simulink library "lib_electric_machine2"  (Simulink 10.1)
settings: Solver=VariableStepAuto  StartTime=0.0  StopTime=10.0  RelTol=1e-3
undefined symbols (not defined in the file or in its folder): amb_tmp, fd_ratio, gb_ratio, gc_inertia, gc_map_spd, gc_map_trq, gc_max_crrnt, gc_max_trq, gc_outpwr_map, gc_overtrq_factor, gc_spd_scale, gc_trq_scale, mc_cp, mc_inertia, mc_init_tmp, mc_inpwr_map, mc_map_spd, mc_map_trq, mc_mass, mc_max_crrnt, mc_max_gen_trq, mc_max_trq, mc_overtrq_factor, mc_sarea, mc_spd_scale, mc_th_calc, mc_trq_scale, mc_tstat, veh_mass, wh_radius
undefined symbols (not defined in the file): logFlag
libraries: lib_electric_machine x1
(part 1 of 3)
settings Model: Creator=sateeshk  LastModifiedBy=sateeshk
settings Model: ModifiedComment=|
  | mokeefe -- Thu Apr 18 08:27:13 2002 -- Version 1.18
  | saving the model:
  | o "without the model browser open"
  | o with only top-level screen visible
  | o with "fit to view" enabled
  | o with "status bar" off and "toolbar" off
  | o with "prompt to update model history with each save" on
settings Model: ModifiedHistory=|
  | mokeefe -- Thu Apr 18 08:27:13 2002 -- Version 1.18
  | saving the model:
  | o "without the model browser open"
  | o with only top-level screen visible
  | o with "fit to view" enabled
  | o with "status bar" off and "toolbar" off
  | o with "prompt to update model history with each save" on
  | 
  | mokeefe -- Thu Apr 18 08:27:13 2002 -- Version 1.18
  | saving the model:
  | o "without the model browser open"
  | o with only top-level screen visible
  | o with "fit to view" enabled
  | o with "status bar" off and "toolbar" off
  | o with "prompt to update model history with each save" on

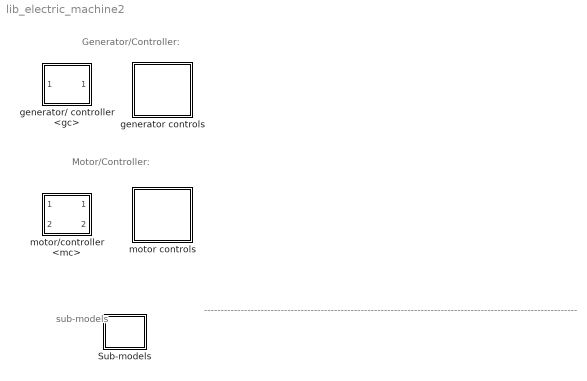
== system lib_electric_machine2 ==
  note: Generator/Controller:
  note: Motor/Controller:
  note: ----------------------------------------------------------------------------------------------------------------
  note: sub-models
  Sub-models : Subsystem
  generator controls : Subsystem
  generator/ controller <gc> : Subsystem  mask(Stand-Alone Generator/Controller Mask){generalName='gc', logPick=Log, initFileName={}, modCell={}, imgFileName='bdi_mc.jpg', DEBUG=OFF}
      mask prompts: generalName "General Name of this Component [char]"; logPick "Log Variables to Workspace?"; initFileName "Initialization File(s) [cell array of char]"; modCell "Modification Cell [2 column cell array of param and val]"; imgFileName "Icon image file name [char--evaluated]"
      mask init:
      | % initialization via m-file script
      | advSACompMaskInit;
      mask TypeOptions logPick: Don't Log | Log
      mask TypeOptions DEBUG: ON | OFF
      mask Display: image(imread(imgFileName))
  motor controls : Subsystem
  motor/controller <mc> : Subsystem  mask(Stand-Alone Motor/Controller Mask){generalName='mc', logPick=Log, initFileName={}, modCell={}, imgFileName='bdi_mc.jpg', DEBUG=OFF}
      mask prompts: generalName "General Name of this Component [char]"; logPick "Log Variables to Workspace?"; initFileName "Initialization File(s) [cell array of char]"; modCell "Modification Cell [2 column cell array of param and val]"; imgFileName "Icon image file name [char--evaluated]"
      mask init:
      | % initialization via m-file script
      | advSACompMaskInit;
      mask TypeOptions logPick: Don't Log | Log
      mask TypeOptions DEBUG: ON | OFF
      mask Display: image(imread(imgFileName))

== system lib_electric_machine2/Sub-models ==
  motor inertia as a function of total vehicle inertia (generous approximation) : Subsystem
  veh mass calc : Subsystem

== system lib_electric_machine2/generator controls ==

== system lib_electric_machine2/generator/ controller <gc> ==
  note: Generator/ CONTROLLER
      | Interface
  "torque and speed supplied to rotor (Nm), (rad/s)" : Inport
  GC Model : Subsystem
  generator output power (W) : Outport  InitialOutput=0
  tag scope: gcReqOut=global, gcSensors=global
  wires:
  "torque and speed supplied to rotor (Nm), (rad/s)"/1 -> GC Model/1("torque and speed supplied to rotor (Nm), (rad/s)")
  [gcControl] -> GC Model/2(Control)
  GC Model/1(requestedOut) -> [gcReqOut]
  GC Model/2(generator output power (W)) -> generator output power (W)/1
  GC Model/3(Sensors) -> [gcSensors]

== system lib_electric_machine2/motor controls ==

== system lib_electric_machine2/motor/controller <mc> ==
  note: MOTOR/ CONTROLLER
      | Interface
  trq and spd out requested : Inport
  electric power in achieved : Inport  Port=2
  motor model & interface : Subsystem
  electric power in  requested : Outport
  "trq and spd out achieved " : Outport  Port=2
  tag scope: mcReqOut=global, mcSensors=global
  wires:
  motor model & interface/4(sensors) -> [mcSensors]
  [mcControl] -> motor model & interface/3(control)
  motor model & interface/1(Out Request) -> [mcReqOut]
  motor model & interface/2(electric power in  requested) -> electric power in  requested/1
  trq and spd out requested/1 -> motor model & interface/1(trq and spd out requested)
  electric power in achieved/1 -> motor model & interface/2(electric power in achieved)
  motor model & interface/3("trq and spd out achieved ") -> "trq and spd out achieved "/1

== system lib_electric_machine2/Sub-models/motor inertia as a function of total vehicle inertia (generous approximation) ==
  gear ratio : Inport
  Product : Product  Inputs=*/  SaturateOnIntegerOverflow=on
  Sum : Sum  Inputs=++|  SaturateOnIntegerOverflow=on
  engine inertia as a fraction of total vehicle inertia  (generous approximation)--denomenator : Fcn  Expr=mc_inertia*u^2
  engine inertia as a fraction of total vehicle inertia  (generous approximation)--numerator : Fcn  Expr=mc_inertia*u^2
  veh mass calc : lib_electric_machine/Sub-models/veh mass calc
      settings: RTWFcnNameOpts=Auto  RTWFileNameOpts=Auto
  Out1 : Outport
  wires:
  engine inertia as a fraction of total vehicle inertia  (generous approximation)--numerator/1 -> Product/1
  Product/1 -> Out1/1
  gear ratio/1 -> engine inertia as a fraction of total vehicle inertia  (generous approximation)--numerator/1, engine inertia as a fraction of total vehicle inertia  (generous approximation)--denomenator/1
  veh mass calc/1 -> Sum/1
  engine inertia as a fraction of total vehicle inertia  (generous approximation)--denomenator/1 -> Sum/2
  Sum/1 -> Product/2

== system lib_electric_machine2/Sub-models/veh mass calc ==
  Constant : Constant  Value=veh_mass
  Sum : Sum  Inputs=|++  SaturateOnIntegerOverflow=on
  Out1 : Outport
  wires:
  [veh_cargo_mass] -> Sum/1
  Constant/1 -> Sum/2
  Sum/1 -> Out1/1

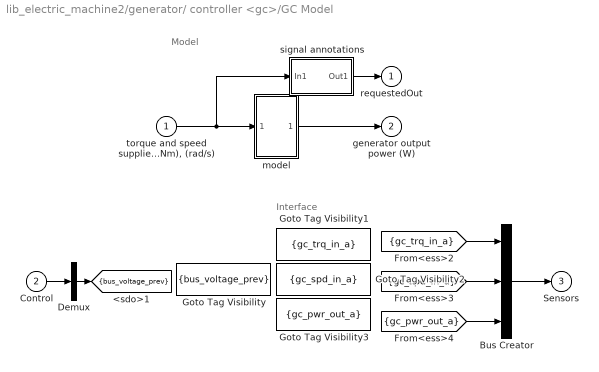
== system lib_electric_machine2/generator/ controller <gc>/GC Model ==
  note: Interface
  note: Model
  "torque and speed supplied to rotor (Nm), (rad/s)" : Inport
  Control : Inport  Port=2
  Bus Creator : BusCreator  Inputs=3
  Demux : Demux  Outputs=1
  Goto Tag Visibility : GotoTagVisibility  GotoTag=bus_voltage_prev
  Goto Tag Visibility1 : GotoTagVisibility  GotoTag=gc_trq_in_a
  Goto Tag Visibility2 : GotoTagVisibility  GotoTag=gc_spd_in_a
  Goto Tag Visibility3 : GotoTagVisibility  GotoTag=gc_pwr_out_a
  model : Subsystem
  signal annotations : Subsystem
  requestedOut : Outport  InitialOutput=0
  generator output power (W) : Outport  Port=2  InitialOutput=0
  Sensors : Outport  Port=3  InitialOutput=0
  tag scope: bus_voltage_prev=scoped
  wires:
  Demux/1 -> [bus_voltage_prev]
  "torque and speed supplied to rotor (Nm), (rad/s)"/1 -> model/1("torque and speed supplied to rotor (Nm), (rad/s)"), signal annotations/1(In1)
  model/1(generator output power (W)) -> generator output power (W)/1
  Control/1 -> Demux/1
  [gc_trq_in_a] -> Bus Creator/1
  [gc_spd_in_a] -> Bus Creator/2
  [gc_pwr_out_a] -> Bus Creator/3
  Bus Creator/1 -> Sensors/1
  signal annotations/1(Out1) -> requestedOut/1

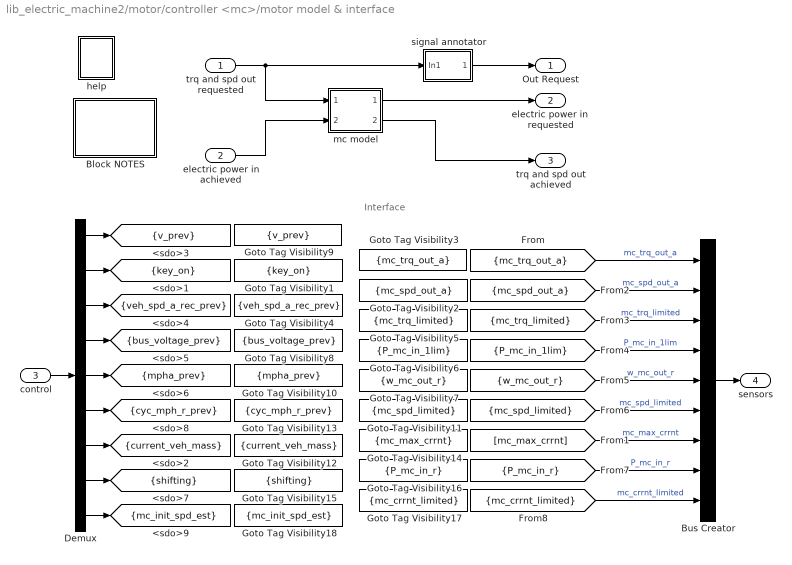
== system lib_electric_machine2/motor/controller <mc>/motor model & interface ==
  note: Interface
  trq and spd out requested : Inport
  electric power in achieved : Inport  Port=2
  control : Inport  Port=3
  Block NOTES : Subsystem
      mask Display: disp('Block\nNOTES')
  Bus Creator : BusCreator  Inputs=9
  Demux : Demux  Outputs=9
  Goto Tag Visibility1 : GotoTagVisibility  GotoTag=key_on
  Goto Tag Visibility10 : GotoTagVisibility  GotoTag=mpha_prev
  Goto Tag Visibility11 : GotoTagVisibility  GotoTag=mc_spd_limited
  Goto Tag Visibility12 : GotoTagVisibility  GotoTag=current_veh_mass
  Goto Tag Visibility13 : GotoTagVisibility  GotoTag=cyc_mph_r_prev
  Goto Tag Visibility14 : GotoTagVisibility  GotoTag=mc_max_crrnt
  Goto Tag Visibility15 : GotoTagVisibility  GotoTag=shifting
  Goto Tag Visibility16 : GotoTagVisibility  GotoTag=P_mc_in_r
  Goto Tag Visibility17 : GotoTagVisibility  GotoTag=mc_crrnt_limited
  Goto Tag Visibility18 : GotoTagVisibility  GotoTag=mc_init_spd_est
  Goto Tag Visibility2 : GotoTagVisibility  GotoTag=mc_spd_out_a
  Goto Tag Visibility3 : GotoTagVisibility  GotoTag=mc_trq_out_a
  Goto Tag Visibility4 : GotoTagVisibility  GotoTag=veh_spd_a_rec_prev
  Goto Tag Visibility5 : GotoTagVisibility  GotoTag=mc_trq_limited
  Goto Tag Visibility6 : GotoTagVisibility  GotoTag=P_mc_in_1lim
  Goto Tag Visibility7 : GotoTagVisibility  GotoTag=w_mc_out_r
  Goto Tag Visibility8 : GotoTagVisibility  GotoTag=bus_voltage_prev
  Goto Tag Visibility9 : GotoTagVisibility  GotoTag=v_prev
  help : Subsystem
      settings: OpenFcn=web(['file:\\\' which('motor_controller.htm')]);
      mask Display: image(imread('doc_man.jpg'))
  mc model : Subsystem
  signal annotator : Subsystem
  Out Request : Outport
  electric power in  requested : Outport  Port=2
  "trq and spd out achieved " : Outport  Port=3
  sensors : Outport  Port=4
  tag scope: bus_voltage_prev=scoped, current_veh_mass=scoped, cyc_mph_r_prev=scoped, key_on=scoped, mc_init_spd_est=scoped, mpha_prev=scoped, shifting=scoped, v_prev=scoped, veh_spd_a_rec_prev=scoped
  wires:
  Demux/9 -> [mc_init_spd_est]
  [mc_crrnt_limited] -> Bus Creator/9  "mc_crrnt_limited"
  [P_mc_in_r] -> Bus Creator/8  "P_mc_in_r"
  Demux/8 -> [shifting]
  trq and spd out requested/1 -> mc model/1("torque and speed  req'd at rotor (Nm), (rad/s)"), signal annotator/1(In1)
  electric power in achieved/1 -> mc model/2(available motor input power (W))
  mc model/1(req'd motor input power (W)) -> electric power in  requested/1
  mc model/2("drive torque and speed avail. at rotor (Nm), (rad/s)") -> "trq and spd out achieved "/1
  Demux/1 -> [v_prev]
  Demux/2 -> [key_on]
  [mc_trq_out_a] -> Bus Creator/1  "mc_trq_out_a"
  [mc_spd_out_a] -> Bus Creator/2  "mc_spd_out_a"
  [mc_trq_limited] -> Bus Creator/3  "mc_trq_limited"
  [P_mc_in_1lim] -> Bus Creator/4  "P_mc_in_1lim"
  [w_mc_out_r] -> Bus Creator/5  "w_mc_out_r"
  Demux/3 -> [veh_spd_a_rec_prev]
  Demux/4 -> [bus_voltage_prev]
  Demux/5 -> [mpha_prev]
  [mc_spd_limited] -> Bus Creator/6  "mc_spd_limited"
  Demux/6 -> [cyc_mph_r_prev]
  Demux/7 -> [current_veh_mass]
  Bus Creator/1 -> sensors/1
  control/1 -> Demux/1
  signal annotator/1(Out1) -> Out Request/1
  [mc_max_crrnt] -> Bus Creator/7  "mc_max_crrnt"

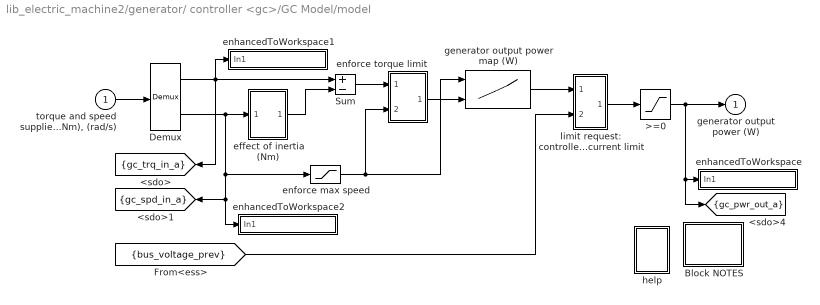
== system lib_electric_machine2/generator/ controller <gc>/GC Model/model ==
  "torque and speed supplied to rotor (Nm), (rad/s)" : Inport
  >=0 : Saturate  UpperLimit=inf  LowerLimit=0
  Block NOTES : Subsystem
      mask Display: disp('Block\nNOTES')
  Demux : Demux  Outputs=2
  Sum : Sum  Inputs=+-  SaturateOnIntegerOverflow=on
  effect of inertia (Nm) : Subsystem
  enforce torque limit : Subsystem
  enforce max speed : Saturate  UpperLimit=max(gc_map_spd)*gc_spd_scale  LowerLimit=0
  enhancedToWorkspace : Subsystem  TreatAsAtomicUnit=on  mask(enhancedToWorkspace){generalName=generalName, specificName=pwr_out_a, logFlag=logFlag}
      mask prompts: generalName "General Name [char-evaluated]"; specificName "Specific Name [char-literal]"; logFlag "Enable flag (1=on,0=off)"
      mask help: A wrapper for the Simulink "To Workspace" block that allows you to evaluate the name of the variable to log to workspace. This is useful to avoid the double logging errors that occur when you pull in two library models that attempt to log to the same variable.
      mask init:
      | enhancedToWsMaker
      settings: CopyFcn=breakLinkCopyFcn  ParentCloseFcn=breakLinkParCloseFcn
      mask Help:
      | <h2>Enhanced To Workspace Block</h2>
      | <h3>Parameters</h3>
      | <UL>
      | <li><b>General Name:</b> This is the more general name of the variable. Variables are saved to the workspace as <i>generalName_specificName</i>. Note that this is an evaluated variable. If you would like to type in the value directly, it must be surrounded with single quotes. Otherwise you can input the name of a variable containing a char string.</li>
      | <li><b>Specific Name:</b> This is the specific name of the variable. Note that this is input as a char literal (i.e., you don't need quotes).</li>
      | <li><b>Enable Flag:</b> This flag should have the value of 0 or 1. If 0, the variable will not be logged to the workspace. If 1, the variable will be logged. This is done so that variable logging can be turned off to improve speed.</li>
      | </ul>
      | <h3>Overview</h3>
      | <p>The enhanced to workspace block was put together to allow one to dynamically resolve variable names at run time in simulink. This is most powerful when used in conjunction with a masked subsystem to allow multiple instances of that masked subsytem to be used in the same model. The strategy is to set the generalName in the block mask which will allow the block to change the general name for all variable logging on the fly.
      | <h3>Helper Files</h3>
      | <p>Three m-files are required by the enhancedToWorkspace block. These files are located in the &lt; ADVISOR root &gt;/GUI directory :
      | <ul>
      | <li><i>enhancedToWsMaker.m</i> This file runs the mask initialization for the block</li>
      | <li><i>breakLinkCopyFcn.m</i> This file is used by the block callback when the simulink block is copied. It is necessary to break the link to the enhancedToWorkspace similar to the To Workspace block in order for it to be able to configure itself. (Try copying simulink's To Workspace block--it is impossible to make a link)</li>
      | <li><i>breakLinkParCloseFcn.m</i> This file is similar to the breakLinkCopyFcn and is used when a parent system is closed</li>
      | </ul>
      | <hr>
      | 
      | <p>Created 2003-Jan-21, Michael Patrick O'Keefe, NREL</p>
      | 
      | <!--
      | <VARDEF>
      | <H3>var_name</H3>
      | <UL>
      | <LI><B>data type</B> data type here</LI>
      | <LI><B>units</B> units here</LI>
      | <LI><B>vehicle type</B> vehicle type here</LI>
      | <LI><B>description</B> description here</LI>
      | </UL>
      | </VARDEF>
      | -->
      mask Display: disp([generalName,'_',specificName])
  enhancedToWorkspace1 : Subsystem  TreatAsAtomicUnit=on  mask(enhancedToWorkspace){generalName=generalName, specificName=trq_in_a, logFlag=logFlag}
      mask prompts: generalName "General Name [char-evaluated]"; specificName "Specific Name [char-literal]"; logFlag "Enable flag (1=on,0=off)"
      mask help: A wrapper for the Simulink "To Workspace" block that allows you to evaluate the name of the variable to log to workspace. This is useful to avoid the double logging errors that occur when you pull in two library models that attempt to log to the same variable.
      mask init:
      | enhancedToWsMaker
      settings: CopyFcn=breakLinkCopyFcn  ParentCloseFcn=breakLinkParCloseFcn
      mask Help:
      | <h2>Enhanced To Workspace Block</h2>
      | <h3>Parameters</h3>
      | <UL>
      | <li><b>General Name:</b> This is the more general name of the variable. Variables are saved to the workspace as <i>generalName_specificName</i>. Note that this is an evaluated variable. If you would like to type in the value directly, it must be surrounded with single quotes. Otherwise you can input the name of a variable containing a char string.</li>
      | <li><b>Specific Name:</b> This is the specific name of the variable. Note that this is input as a char literal (i.e., you don't need quotes).</li>
      | <li><b>Enable Flag:</b> This flag should have the value of 0 or 1. If 0, the variable will not be logged to the workspace. If 1, the variable will be logged. This is done so that variable logging can be turned off to improve speed.</li>
      | </ul>
      | <h3>Overview</h3>
      | <p>The enhanced to workspace block was put together to allow one to dynamically resolve variable names at run time in simulink. This is most powerful when used in conjunction with a masked subsystem to allow multiple instances of that masked subsytem to be used in the same model. The strategy is to set the generalName in the block mask which will allow the block to change the general name for all variable logging on the fly.
      | <h3>Helper Files</h3>
      | <p>Three m-files are required by the enhancedToWorkspace block. These files are located in the &lt; ADVISOR root &gt;/GUI directory :
      | <ul>
      | <li><i>enhancedToWsMaker.m</i> This file runs the mask initialization for the block</li>
      | <li><i>breakLinkCopyFcn.m</i> This file is used by the block callback when the simulink block is copied. It is necessary to break the link to the enhancedToWorkspace similar to the To Workspace block in order for it to be able to configure itself. (Try copying simulink's To Workspace block--it is impossible to make a link)</li>
      | <li><i>breakLinkParCloseFcn.m</i> This file is similar to the breakLinkCopyFcn and is used when a parent system is closed</li>
      | </ul>
      | <hr>
      | 
      | <p>Created 2003-Jan-21, Michael Patrick O'Keefe, NREL</p>
      | 
      | <!--
      | <VARDEF>
      | <H3>var_name</H3>
      | <UL>
      | <LI><B>data type</B> data type here</LI>
      | <LI><B>units</B> units here</LI>
      | <LI><B>vehicle type</B> vehicle type here</LI>
      | <LI><B>description</B> description here</LI>
      | </UL>
      | </VARDEF>
      | -->
      mask Display: disp([generalName,'_',specificName])
  enhancedToWorkspace2 : Subsystem  TreatAsAtomicUnit=on  mask(enhancedToWorkspace){generalName=generalName, specificName=spd_in_a, logFlag=logFlag}
      mask prompts: generalName "General Name [char-evaluated]"; specificName "Specific Name [char-literal]"; logFlag "Enable flag (1=on,0=off)"
      mask help: A wrapper for the Simulink "To Workspace" block that allows you to evaluate the name of the variable to log to workspace. This is useful to avoid the double logging errors that occur when you pull in two library models that attempt to log to the same variable.
      mask init:
      | enhancedToWsMaker
      settings: CopyFcn=breakLinkCopyFcn  ParentCloseFcn=breakLinkParCloseFcn
      mask Help:
      | <h2>Enhanced To Workspace Block</h2>
      | <h3>Parameters</h3>
      | <UL>
      | <li><b>General Name:</b> This is the more general name of the variable. Variables are saved to the workspace as <i>generalName_specificName</i>. Note that this is an evaluated variable. If you would like to type in the value directly, it must be surrounded with single quotes. Otherwise you can input the name of a variable containing a char string.</li>
      | <li><b>Specific Name:</b> This is the specific name of the variable. Note that this is input as a char literal (i.e., you don't need quotes).</li>
      | <li><b>Enable Flag:</b> This flag should have the value of 0 or 1. If 0, the variable will not be logged to the workspace. If 1, the variable will be logged. This is done so that variable logging can be turned off to improve speed.</li>
      | </ul>
      | <h3>Overview</h3>
      | <p>The enhanced to workspace block was put together to allow one to dynamically resolve variable names at run time in simulink. This is most powerful when used in conjunction with a masked subsystem to allow multiple instances of that masked subsytem to be used in the same model. The strategy is to set the generalName in the block mask which will allow the block to change the general name for all variable logging on the fly.
      | <h3>Helper Files</h3>
      | <p>Three m-files are required by the enhancedToWorkspace block. These files are located in the &lt; ADVISOR root &gt;/GUI directory :
      | <ul>
      | <li><i>enhancedToWsMaker.m</i> This file runs the mask initialization for the block</li>
      | <li><i>breakLinkCopyFcn.m</i> This file is used by the block callback when the simulink block is copied. It is necessary to break the link to the enhancedToWorkspace similar to the To Workspace block in order for it to be able to configure itself. (Try copying simulink's To Workspace block--it is impossible to make a link)</li>
      | <li><i>breakLinkParCloseFcn.m</i> This file is similar to the breakLinkCopyFcn and is used when a parent system is closed</li>
      | </ul>
      | <hr>
      | 
      | <p>Created 2003-Jan-21, Michael Patrick O'Keefe, NREL</p>
      | 
      | <!--
      | <VARDEF>
      | <H3>var_name</H3>
      | <UL>
      | <LI><B>data type</B> data type here</LI>
      | <LI><B>units</B> units here</LI>
      | <LI><B>vehicle type</B> vehicle type here</LI>
      | <LI><B>description</B> description here</LI>
      | </UL>
      | </VARDEF>
      | -->
      mask Display: disp([generalName,'_',specificName])
  generator output power map (W) : Lookup2D  RowIndex=gc_map_spd*gc_spd_scale  ColumnIndex=gc_map_trq*gc_trq_scale  Table=gc_outpwr_map*gc_spd_scale*gc_trq_scale  SaturateOnIntegerOverflow=on  InputSameDT=on
  help : Subsystem
      settings: OpenFcn=web(['file:\\\' which('generator_controller.htm')]);
      mask Display: image(imread('doc_man.jpg'))
  limit request: controller current limit : Subsystem
  generator output power (W) : Outport  InitialOutput=0
  tag scope: gc_pwr_out_a=scoped, gc_spd_in_a=scoped, gc_trq_in_a=scoped
  wires:
  >=0/1 -> generator output power (W)/1, enhancedToWorkspace/1(In1), [gc_pwr_out_a]
  limit request: controller current limit/1(out_1) -> >=0/1
  Demux/1 -> Sum/1, [gc_trq_in_a], enhancedToWorkspace1/1(In1)
  [bus_voltage_prev] -> limit request: controller current limit/2(bus voltage (V))
  enforce max speed/1 -> generator output power map (W)/1, enforce torque limit/2(limited generator speed (rad/s))
  generator output power map (W)/1 -> limit request: controller current limit/1(computed output power (W))
  Sum/1 -> enforce torque limit/1(req'd generator input torque (Nm))
  enforce torque limit/1(limited generator input torque (Nm)) -> generator output power map (W)/2
  effect of inertia (Nm)/1(out_1) -> Sum/2
  "torque and speed supplied to rotor (Nm), (rad/s)"/1 -> Demux/1
  Demux/2 -> effect of inertia (Nm)/1(in_1), enforce max speed/1, [gc_spd_in_a], enhancedToWorkspace2/1(In1)

== system lib_electric_machine2/generator/ controller <gc>/GC Model/signal annotations ==
  In1 : Inport
  Bus Creator : BusCreator  Inputs=2
  Demux : Demux  Outputs=2
  Out1 : Outport
  wires:
  In1/1 -> Demux/1
  Bus Creator/1 -> Out1/1
  Demux/1 -> Bus Creator/1  "gc_trq_in_a"
  Demux/2 -> Bus Creator/2  "gc_spd_in_a"

== system lib_electric_machine2/motor/controller <mc>/motor model & interface/Block NOTES ==
  note: Available torque is computed from available power by assuming that the ratio of rotor torque to input
      | (electric) power is the same for the actual/achievable situation as was computed for the request.  This
      | is mathematically equivalent to assuming that the motor/controller efficiency.  Rotor speed for the
      | actual/achievable calculations is as computed in the 'request' branch.
  note: This motor/controller model includes loss data, rotational inertia, and performance limits.
  note: Note: The block interface will auto-configure itself based upon the generalName variable set in
      | the subsystem component mask. The user must connect and create/configure the control block
      | up correctly based upon the control (nControl), sensor (nSensors), and requested out signals (nReqOut).

== system lib_electric_machine2/motor/controller <mc>/motor model & interface/help ==
